simulink subsystem "LQR"  (R2024a)
settings: Solver=VariableStepAuto  StartTime=0.0  StopTime=10.0  RelTol=1e-3
undefined symbols (not defined in the file): K_LQR, u_eq, x_eq
settings Model: Creator=Bocchio  LastModifiedBy=Bocchio

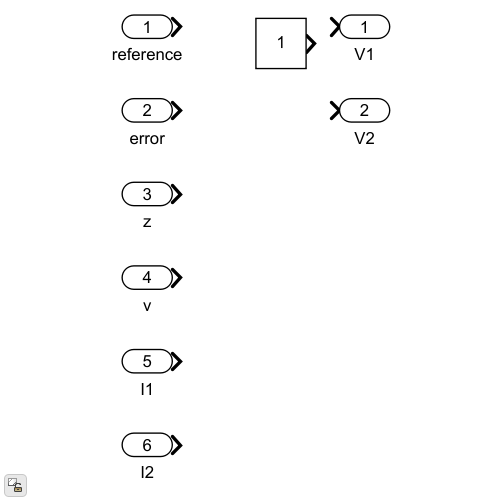
[thumbnail: Simulink's stored preview of the top-level diagram]
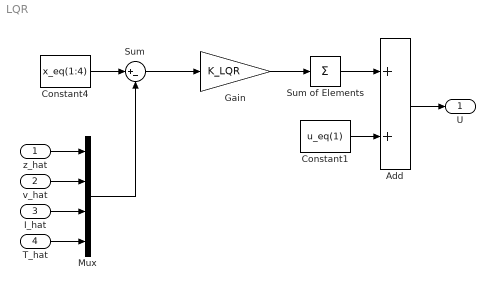
== system LQR ==
  z_hat : Inport
  v_hat : Inport  Port=2
  I_hat : Inport  Port=3
  T_hat : Inport  Port=4
  Add : Sum
  Constant1 : Constant  Value=u_eq(1)
  Constant4 : Constant  Value=x_eq(1:4)
  Gain : Gain  Gain=K_LQR
  Mux : Mux
  Sum : Sum  Inputs=|+-
  Sum of Elements : Sum  Inputs=+  CollapseDim=2
  U : Outport
  wires:
  Gain/1 -> Sum of Elements/1
  Constant1/1 -> Add/2
  z_hat/1 -> Mux/1
  v_hat/1 -> Mux/2
  I_hat/1 -> Mux/3
  Constant4/1 -> Sum/1
  Mux/1 -> Sum/2
  Sum/1 -> Gain/1
  Sum of Elements/1 -> Add/1
  Add/1 -> U/1
  T_hat/1 -> Mux/4
